simulink model "fuelsys_LN2_breach"  (R2017a)
settings: Solver=ode45  StartTime=0.0  StopTime=tspan(end)  FixedStep=0.001  RelTol=1e-5  AbsTol=1e-6
PostLoadFcn:
  | sldemo_fuelsys_data(bdroot,'initialize_data','orig','float');
model workspace (MAT data in the model file):
  PressEst = [0.806253176324 0.553142316929 0.37151500209 0.277667903103 0.220198954207 0.181288665766 0.153200000489 0.115431020872 0.0913067476324 0.0746519188607 0.0625231108324 0.0533383634277 ... (306 elements, 18x17)]
  PressVect = [0.05 0.1 0.15 0.2 0.25 0.3 0.35 0.4 0.45 0.5 0.55 0.6 0.65 0.7 0.75 0.8 0.85 0.9 0.95]
  PumpCon = [-0.0556348 -0.0022828 0.0256932 0.0435188 0.0562692 0.0661194857143 0.0741572 0.08697 0.0972452 0.106070342857 0.1139892 0.121303866667 ... (342 elements, 18x19)]
  RampRateKiX = [100 200 300 400 500 600]
  RampRateKiY = [0 0.2 0.4 0.6 0.8 1]
  RampRateKiZ = [0.012  0.024  0.036  0.048  0.06  0.072; 0.024  0.048  0.072  0.096  0.12  0.144; 0.036  0.072  0.108  0.144  0.18  0.216; 0.048  0.096  0.144  0.192  0.24  0.288; 0.06  0.12  0.18  0.24  0.3  0.36; 0.072  0.144  0.216  0.288  0.36  0.432]
  SpeedEst = [471.837839721 550.80940091 777.559313277 1080.9243499 1418.36795322 1769.7468768 2125.37309264 2480.20345067 2831.37796793 3177.14006959 3516.32917143 4064.90417867 ... (323 elements, 17x19)]
  SpeedVect = [50 75 100 125 150 175 200 250 300 350 400 450 500 600 700 800 900 1000]
  ThrotEst = [0 0 0 0 0 0 0 0 0 0 0 0 ... (342 elements, 18x19)]
  ThrotVect = [0 3 6 9 12 15 18 21 24 27 30 35 46 57 68 79 90]
  ego_sw = 1
  engine_speed = 300
  hys = 25
  map_sw = 1
  max_ego = 1.2
  max_press = 0.95
  max_speed = 628
  max_throt = 90
  min_press = 0.05
  min_speed = 50
  min_throt = 3
  speed_sw = 1
  st_range = 0.0001
  throttle_sw = 1
  zero_thresh = 250
undefined symbols (not defined in the file): DiscIntNeverNeededParam, sld_FuelModes, sldvsubsys
libraries: simulink x7, simulink_extras x2
(part 1 of 2)
CloseFcn:
  | clear EngSensors u8En* s16En* sldemo_fuelsys_output
Description:
  | This is a model of a fuel control system where Stateflow(R) is used to handle the fault management of the system.
  | The system contains four separate sensors: a throttle sensor, a speed sensor, an oxygen sensor, and a pressure sensor.
  | Each of these sensors is represented by a parallel state in Stateflow.  Each parallel state contains two substates, a
  | normal state and a failed state (the exception being the oxygen sensor, which also contains a warmup state).
  | 
  | If any of the sensor readings is outside an acceptable range, then a fault is registered in Stateflow, and the
  | substate of the corresponding subsystem transitions to the failed state.  If a subsystem recovers, it can
  | transition back to the normal state.  The number of failures in the system at any given time is represented
  | in the Fail parallel state.
  | 
  | The last parallel state in the Stateflow chart is called Fueling_Mode.  This state regulates the oxygen to
  | fuel mixture ratio.  If a failure is detected, then the oxygen to fuel ratio is increased.  If multiple failures
  | are detected, then the fuel system is disabled until there are no longer multiple failures in the system.
settings Model: ModifiedByFormat=The MathWorks Inc.  ExtModeTrigMode=oneshot  ExtModeArmWhenConnect=off  ExtModeAutoUpdateStatusClock=off  Creator=The MathWorks, Inc.  LastModifiedBy=The MathWorks Inc.
settings DataIOCC: ExternalInput=[t__, u__]  LoadExternalInput=on  SaveFormat=StructureWithTime  ReturnWorkspaceOutputs=on
settings OptimizationCC: DefaultParameterBehavior=Inlined  UseDivisionForNetSlopeComputation=UseDivisionForReciprocalsOfIntegersOnly  InlineInvariantSignals=on  EnhancedBackFolding=on  StrengthReduction=on  BooleansAsBitfields=on  PassReuseOutputArgsAs=Individual arguments  ExpressionDepthLimit=2147483647  ZeroExternalMemoryAtStartup=off  ZeroInternalMemoryAtStartup=off  NoFixptDivByZeroProtection=on  EfficientFloat2IntCast=on  LifeSpan=1
settings DebuggingCC: SignalInfNanChecking=error  SaveWithParameterizedLinksMsg=none  UnderspecifiedInitializationDetection=Classic  CheckExecutionContextPreStartOutputMsg=on  CheckExecutionContextRuntimeOutputMsg=on  IntegerOverflowMsg=none  ParameterDowncastMsg=warning  ParameterOverflowMsg=none  ParameterPrecisionLossMsg=none  UnderSpecifiedDataTypeMsg=warning  FcnCallInpInsideContextMsg=warning  UniqueDataStoreMsg=error  BusObjectLabelMismatch=error  StateNameClashWarn=warning  StrictBusMsg=ErrorOnBusTreatedAsVector  SFUnexpectedBacktrackingDiag=warning  SFNoUnconditionalDefaultTransitionDiag=warning  SFExecutionAtInitializationDiag=none  IntegerSaturationMsg=none
settings HardwareCC: ProdBitPerPointer=32  ProdBitPerSizeT=32  ProdBitPerPtrDiffT=32  ProdLargestAtomicFloat=None  ProdWordSize=32  ProdHWDeviceType=Specified
settings ModelReferenceCC: PropagateSignalLabelsOutOfModel=off
settings SFSimCC: SimParseCustomCode=off  MATLABDynamicMemAlloc=off
settings RTWCC: SystemTargetFile=ert.tlc  TemplateMakefile=ert_default_tmf  Description=Real-Time Workshop Embedded Coder  RTWVerbose=off  IncludeHyperlinkInReport=on
settings CodeAppCC: ForceParamTrailComments=on  IgnoreCustomStorageClasses=off  IgnoreTestpoints=on  SimulinkDataObjDesc=on  SFDataObjDesc=on  CustomSymbolStrGlobalVar=rt$N$M  CustomSymbolStrType=$N$M  CustomSymbolStrFcn=$N$M$F  CustomSymbolStrMacro=$N$M  InsertBlockDesc=on  InternalIdentifier=Classic  ReqsInCode=on
settings ERTTargetCC: MultiwordLength=2048  GenerateSampleERTMain=on  IncludeMdlTerminateFcn=off  SupportAbsoluteTime=off  SupportNonFinite=off  SupportComplex=off  InlinedParameterPlacement=NonHierarchical  ERTCustomFileTemplate=example_file_process.tlc  ConvertIfToSwitch=off  SuppressUnreachableDefaultCases=off
settings ConfigComp: CovScope=Subsystem  CovPath=/fuel_rate_control/control_logic  CovMetricSettings=dw  CovHtmlReporting=on  CovSaveCumulativeToWorkspaceVar=on  CovSaveSingleToWorkspaceVar=on  CovExternalEMLEnable=off  CovSFcnEnable=off

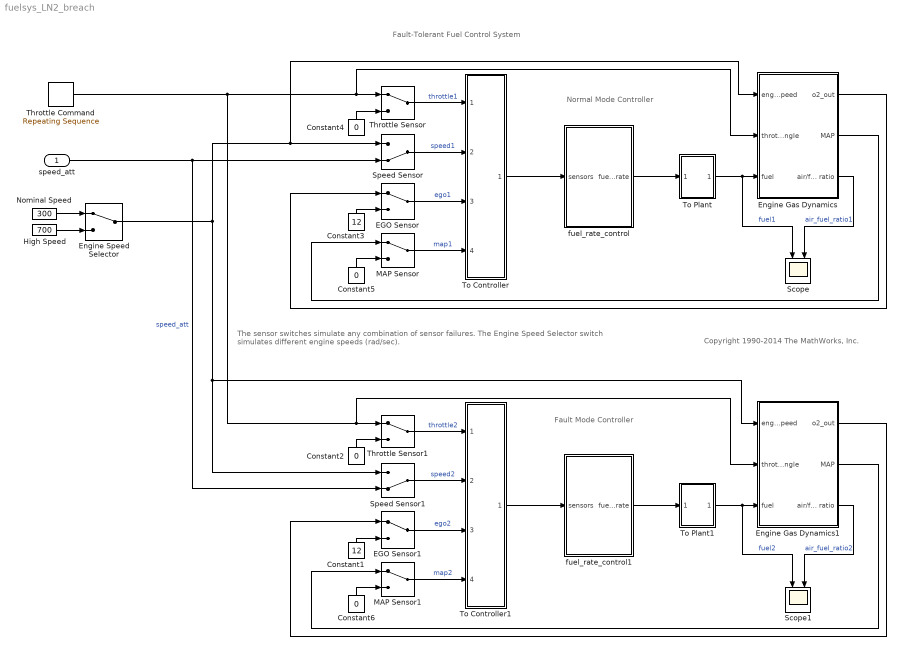
== system fuelsys_LN2_breach ==
  note: Normal Mode Controller
  note: Fault-Tolerant Fuel Control System
  note: Copyright 1990-2014 The MathWorks, Inc.
  note: The sensor switches simulate any combination of sensor failures.
      | The Engine Speed Selector switch simulates different engine speeds (rad/sec).
  note: Fault Mode Controller
  speed_att : Inport
  Constant1 : Constant  Value=12
  Constant{2,4..6} (4 alike) : Constant  Value=0
  Constant3 : Constant  Value=12
  EGO Sensor : ManualSwitch
  EGO Sensor1 : ManualSwitch
  Engine Speed Selector : ManualSwitch
  Engine Gas Dynamics : Subsystem
  Engine Gas Dynamics1 : Subsystem
  High Speed : Constant  Value=700
  MAP Sensor : ManualSwitch
  MAP Sensor1 : ManualSwitch
  Nominal Speed : Constant  Value=300
  Scope : Scope  NumInputPorts=2
  Scope1 : Scope  NumInputPorts=2
  Speed Sensor : ManualSwitch  CurrentSetting=0
  Speed Sensor1 : ManualSwitch  CurrentSetting=0
  Throttle Command : simulink/Sources/Repeating Sequence  rep_seq_t=[0 2 4]  rep_seq_y=[10 20 10]
  Throttle Sensor : ManualSwitch
  Throttle Sensor1 : ManualSwitch
  To Controller : Subsystem
      mask Display: fprintf('Convert')
  To Controller1 : Subsystem
      mask Display: fprintf('Convert')
  To Plant : Subsystem
      mask Display: fprintf('Convert')
  To Plant1 : Subsystem
      mask Display: fprintf('Convert')
  fuel_rate_control : Subsystem  Tag=FuelRateControl  TreatAsAtomicUnit=on
  fuel_rate_control1 : Subsystem  Tag=FuelRateControl  TreatAsAtomicUnit=on
  wires:
  Engine Gas Dynamics/3(air/fuel ratio) -> Scope/2  "air_fuel_ratio1"
  fuel_rate_control/1(fuel_rate) -> To Plant/1(In1)
  Engine Gas Dynamics/1(o2_out) -> EGO Sensor/1
  Constant5/1 -> MAP Sensor/2
  Constant3/1 -> EGO Sensor/2
  Constant4/1 -> Throttle Sensor/2
  Engine Gas Dynamics/2(MAP) -> MAP Sensor/1
  High Speed/1 -> Engine Speed Selector/2
  Nominal Speed/1 -> Engine Speed Selector/1
  EGO Sensor/1 -> To Controller/3(ego)  "ego1"
  MAP Sensor/1 -> To Controller/4(map)  "map1"
  Throttle Sensor/1 -> To Controller/1(throttle)  "throttle1"
  Speed Sensor/1 -> To Controller/2(speed)  "speed1"
  To Plant/1(Out1) -> Scope/1, Engine Gas Dynamics/3(fuel)  "fuel1"
  To Controller/1(sensors) -> fuel_rate_control/1(sensors)
  Engine Gas Dynamics1/3(air/fuel ratio) -> Scope1/2  "air_fuel_ratio2"
  Engine Speed Selector/1 -> Engine Gas Dynamics/1(engine speed), Speed Sensor/1, Engine Gas Dynamics1/1(engine speed), Speed Sensor1/1
  fuel_rate_control1/1(fuel_rate) -> To Plant1/1(In1)
  Engine Gas Dynamics1/1(o2_out) -> EGO Sensor1/1
  Constant6/1 -> MAP Sensor1/2
  Constant1/1 -> EGO Sensor1/2
  Throttle Command/1 -> Engine Gas Dynamics/2(throttle angle), Throttle Sensor/1, Engine Gas Dynamics1/2(throttle angle), Throttle Sensor1/1
  Constant2/1 -> Throttle Sensor1/2
  Engine Gas Dynamics1/2(MAP) -> MAP Sensor1/1
  EGO Sensor1/1 -> To Controller1/3(ego)  "ego2"
  MAP Sensor1/1 -> To Controller1/4(map)  "map2"
  Throttle Sensor1/1 -> To Controller1/1(throttle)  "throttle2"
  Speed Sensor1/1 -> To Controller1/2(speed)  "speed2"
  To Plant1/1(Out1) -> Scope1/1, Engine Gas Dynamics1/3(fuel)  "fuel2"
  To Controller1/1(sensors) -> fuel_rate_control1/1(sensors)
  speed_att/1 -> Speed Sensor1/2, Speed Sensor/2  "speed_att"

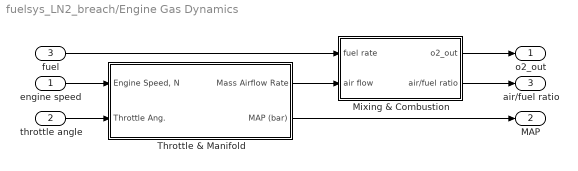
== system fuelsys_LN2_breach/Engine Gas Dynamics ==
  engine speed : Inport
  throttle angle : Inport  Port=2
  fuel : Inport  Port=3
  Mixing & Combustion : Subsystem
  Throttle & Manifold : Subsystem
  o2_out : Outport
  MAP : Outport  Port=2
  air/fuel ratio : Outport  Port=3
  wires:
  Throttle & Manifold/1(Mass Airflow Rate) -> Mixing & Combustion/2(air flow)
  fuel/1 -> Mixing & Combustion/1(fuel rate)
  engine speed/1 -> Throttle & Manifold/1("Engine Speed, N")
  throttle angle/1 -> Throttle & Manifold/2(Throttle Ang.)
  Mixing & Combustion/2(air/fuel ratio) -> air/fuel ratio/1
  Throttle & Manifold/2(MAP (bar)) -> MAP/1
  Mixing & Combustion/1(o2_out) -> o2_out/1

== system fuelsys_LN2_breach/Engine Gas Dynamics1 ==
  engine speed : Inport
  throttle angle : Inport  Port=2
  fuel : Inport  Port=3
  Mixing & Combustion : Subsystem
  Throttle & Manifold : Subsystem
  o2_out : Outport
  MAP : Outport  Port=2
  air/fuel ratio : Outport  Port=3
  wires:
  Throttle & Manifold/1(Mass Airflow Rate) -> Mixing & Combustion/2(air flow)
  fuel/1 -> Mixing & Combustion/1(fuel rate)
  engine speed/1 -> Throttle & Manifold/1("Engine Speed, N")
  throttle angle/1 -> Throttle & Manifold/2(Throttle Ang.)
  Mixing & Combustion/2(air/fuel ratio) -> air/fuel ratio/1
  Throttle & Manifold/2(MAP (bar)) -> MAP/1
  Mixing & Combustion/1(o2_out) -> o2_out/1

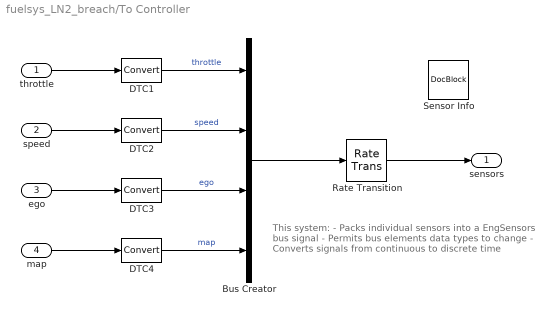
== system fuelsys_LN2_breach/To Controller ==
  note: This system:
      | - Packs individual sensors into a EngSensors bus signal
      | - Permits bus elements data types to change
      | - Converts signals from continuous to discrete time
  throttle : Inport
  speed : Inport  Port=2
  ego : Inport  Port=3
  map : Inport  Port=4
  Bus Creator : BusCreator  Inputs=4  OutDataTypeStr=Bus: EngSensors  NonVirtualBus=on
  DTC{1..4} (4 alike) : DataTypeConversion  SampleTime=[0 1]
  Rate Transition : RateTransition  OutPortSampleTime=0.01
  Sensor Info : simulink/Model-Wide Utilities/DocBlock  DocumentType=Text
      content=|
      | Measurement Descriptions
      | ========================
      |
      | Throttle Angle (degrees):
      | min=3, max=90, precision=0.1
      |
      | Engine Speed (radians/sec.):
      | min=0, max=620, precision=.1
      |
      | Ego Sensor (volts):
      | min=0, max=12, precision=.05
      |
      | Manifold Pressure (bar):
      | min=0.001, max=1, precision=.001
  sensors : Outport
  wires:
  throttle/1 -> DTC1/1
  DTC1/1 -> Bus Creator/1  "throttle"
  speed/1 -> DTC2/1
  DTC2/1 -> Bus Creator/2  "speed"
  ego/1 -> DTC3/1
  DTC3/1 -> Bus Creator/3  "ego"
  map/1 -> DTC4/1
  DTC4/1 -> Bus Creator/4  "map"
  Bus Creator/1 -> Rate Transition/1
  Rate Transition/1 -> sensors/1

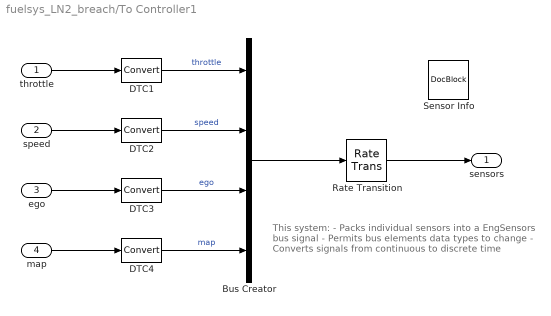
== system fuelsys_LN2_breach/To Controller1 ==
  note: This system:
      | - Packs individual sensors into a EngSensors bus signal
      | - Permits bus elements data types to change
      | - Converts signals from continuous to discrete time
  throttle : Inport
  speed : Inport  Port=2
  ego : Inport  Port=3
  map : Inport  Port=4
  Bus Creator : BusCreator  Inputs=4  OutDataTypeStr=Bus: EngSensors  NonVirtualBus=on
  DTC{1..4} (4 alike) : DataTypeConversion  SampleTime=[0 1]
  Rate Transition : RateTransition  OutPortSampleTime=0.01
  Sensor Info : simulink/Model-Wide Utilities/DocBlock  DocumentType=Text
      content=|
      | Measurement Descriptions
      | ========================
      |
      | Throttle Angle (degrees):
      | min=3, max=90, precision=0.1
      |
      | Engine Speed (radians/sec.):
      | min=0, max=620, precision=.1
      |
      | Ego Sensor (volts):
      | min=0, max=12, precision=.05
      |
      | Manifold Pressure (bar):
      | min=0.001, max=1, precision=.001
  sensors : Outport
  wires:
  throttle/1 -> DTC1/1
  DTC1/1 -> Bus Creator/1  "throttle"
  speed/1 -> DTC2/1
  DTC2/1 -> Bus Creator/2  "speed"
  ego/1 -> DTC3/1
  DTC3/1 -> Bus Creator/3  "ego"
  map/1 -> DTC4/1
  DTC4/1 -> Bus Creator/4  "map"
  Bus Creator/1 -> Rate Transition/1
  Rate Transition/1 -> sensors/1

== system fuelsys_LN2_breach/To Plant ==
  note: This system:
      | - Permits upstream signal data type to change
      | - Converts signals from discrete to continuous time
  In1 : Inport
  DTC5 : DataTypeConversion
  Rate Transition1 : RateTransition  Integrity=off  X0=1.6  OutPortSampleTime=0
  Out1 : Outport
  wires:
  DTC5/1 -> Rate Transition1/1
  In1/1 -> DTC5/1
  Rate Transition1/1 -> Out1/1

== system fuelsys_LN2_breach/To Plant1 ==
  note: This system:
      | - Permits upstream signal data type to change
      | - Converts signals from discrete to continuous time
  In1 : Inport
  DTC5 : DataTypeConversion
  Rate Transition1 : RateTransition  Integrity=off  X0=1.6  OutPortSampleTime=0
  Out1 : Outport
  wires:
  DTC5/1 -> Rate Transition1/1
  In1/1 -> DTC5/1
  Rate Transition1/1 -> Out1/1

== system fuelsys_LN2_breach/fuel_rate_control ==
  note: Fuel Rate Control Subsystem
  sensors : Inport  OutDataTypeStr=Bus: EngSensors
  Bus Selector1 : BusSelector  OutputSignals=speed
  airflow_calc : Subsystem
  control_logic : Stateflow chart  Description=Stateflow diagram to determine control system operating mode  TreatAsAtomicUnit=on
  fuel_calc : Subsystem
  validate_sample_time : Subsystem  Tag=VerificationSubsystem  DisableCoverage=on  LoadFcn=sldvsubsys('check')  TreatAsAtomicUnit=on  SimViewingDevice=on  mask(VerificationSubsystem){}
      mask init:
      | sldvsubsys('maskInit');
      settings: CopyFcn=sldvsubsys('copy');  OpenFcn=open_system(gcb,'force');
      settings: PreSaveFcn=|
      | set_param(gcb,'SimViewingDevice','on');
      | sldvsubsys('check');
      mask Help: helpview(fullfile(docroot,'toolbox','sldv','sldv.map'),'verificationsubsystem')
      mask Display: image(imread('sldvicon_versubsys.png','BackGroundColor',[1 1 1]),'center');
  fuel_rate : Outport
  wires:
  fuel_calc/1(fuel_rate) -> fuel_rate/1
  airflow_calc/1(est_airflow) -> fuel_calc/1(est_airflow)
  sensors/1 -> control_logic/1(es_i), Bus Selector1/1
  control_logic/3(fuel_mode) -> airflow_calc/3(fuel_mode), fuel_calc/3(fuel_mode)
  control_logic/1(es_o) -> airflow_calc/1(sensors)
  control_logic/2(" O2_normal") -> airflow_calc/2(O2_normal)
  airflow_calc/2(fb_correction) -> fuel_calc/2(fb_correction)
  Bus Selector1/1 -> validate_sample_time/1(In1)  "<speed>"

== system fuelsys_LN2_breach/fuel_rate_control1 ==
  note: Fuel Rate Control Subsystem
  sensors : Inport  OutDataTypeStr=Bus: EngSensors
  Bus Selector1 : BusSelector  OutputSignals=speed
  airflow_calc : Subsystem
  control_logic : Stateflow chart  Description=Stateflow diagram to determine control system operating mode  TreatAsAtomicUnit=on
  fuel_calc : Subsystem
  validate_sample_time : Subsystem  Tag=VerificationSubsystem  DisableCoverage=on  LoadFcn=sldvsubsys('check')  TreatAsAtomicUnit=on  SimViewingDevice=on  mask(VerificationSubsystem){}
      mask init:
      | sldvsubsys('maskInit');
      settings: CopyFcn=sldvsubsys('copy');  OpenFcn=open_system(gcb,'force');
      settings: PreSaveFcn=|
      | set_param(gcb,'SimViewingDevice','on');
      | sldvsubsys('check');
      mask Help: helpview(fullfile(docroot,'toolbox','sldv','sldv.map'),'verificationsubsystem')
      mask Display: image(imread('sldvicon_versubsys.png','BackGroundColor',[1 1 1]),'center');
  fuel_rate : Outport
  wires:
  fuel_calc/1(fuel_rate) -> fuel_rate/1
  airflow_calc/1(est_airflow) -> fuel_calc/1(est_airflow)
  sensors/1 -> control_logic/1(es_i), Bus Selector1/1
  control_logic/3(fuel_mode) -> airflow_calc/3(fuel_mode), fuel_calc/3(fuel_mode)
  control_logic/1(es_o) -> airflow_calc/1(sensors)
  control_logic/2(" O2_normal") -> airflow_calc/2(O2_normal)
  airflow_calc/2(fb_correction) -> fuel_calc/2(fb_correction)
  Bus Selector1/1 -> validate_sample_time/1(In1)  "<speed>"

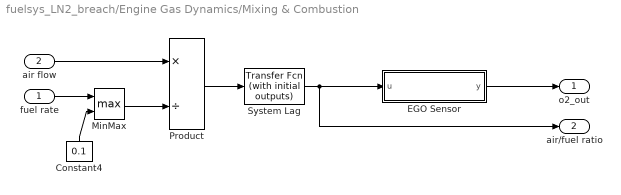
== system fuelsys_LN2_breach/Engine Gas Dynamics/Mixing & Combustion ==
  fuel rate : Inport
  air flow : Inport  Port=2
  Constant4 : Constant  Value=0.1
  EGO Sensor : MATLAB Function  TreatAsAtomicUnit=on
  MinMax : MinMax  Function=max  Inputs=2  SaturateOnIntegerOverflow=on  InputSameDT=on
  Product : Product  Inputs=*/  SaturateOnIntegerOverflow=on  RndMeth=Zero  InputSameDT=on  OutDataTypeStr=Inherit: Same as first input
  System Lag : simulink_extras/Additional Linear/Transfer Fcn (with initial outputs)  N=3  D=[1 3]  Y0=1/14.6  U0=1/14.6
  o2_out : Outport
  air/fuel ratio : Outport  Port=2
  wires:
  Constant4/1 -> MinMax/2
  fuel rate/1 -> MinMax/1
  MinMax/1 -> Product/2
  Product/1 -> System Lag/1
  System Lag/1 -> air/fuel ratio/1, EGO Sensor/1(u)
  EGO Sensor/1(y) -> o2_out/1
  air flow/1 -> Product/1

== system fuelsys_LN2_breach/Engine Gas Dynamics/Throttle & Manifold ==
  note: Air-Fuel Intake Dynamics
  "Engine Speed, N" : Inport
  Throttle Ang. : Inport  Port=2
  "Atmospheric Pressure, Pa (bar)" : Constant  Value=1.0
  Intake Manifold : Subsystem
  Limit to Positive : Saturate  UpperLimit=inf  LowerLimit=0
  Throttle : Subsystem
  Mass Airflow Rate : Outport
  MAP (bar) : Outport  Port=2
  wires:
  Limit to Positive/1 -> Throttle/1("Throttle Angle, theta (deg)")
  Throttle Ang./1 -> Limit to Positive/1
  Throttle/1("Throttle Flow, mdot (g/s)") -> Intake Manifold/1(mdot Input (g/s))
  "Engine Speed, N"/1 -> Intake Manifold/2(N (rad/sec))
  Intake Manifold/1(mdot to Cylinder (g/s)) -> Mass Airflow Rate/1
  "Atmospheric Pressure, Pa (bar)"/1 -> Throttle/3("Atmospheric Pressure, Pa (bar) ")
  Intake Manifold/2("Manifold Pressure, Pm (bar)") -> Throttle/2("Manifold Pressure, Pm (bar)"), MAP (bar)/1

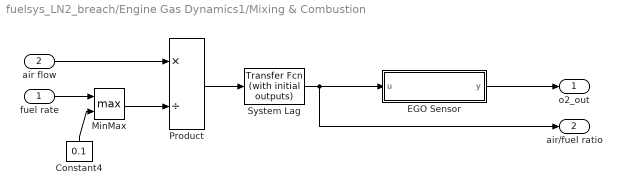
== system fuelsys_LN2_breach/Engine Gas Dynamics1/Mixing & Combustion ==
  fuel rate : Inport
  air flow : Inport  Port=2
  Constant4 : Constant  Value=0.1
  EGO Sensor : MATLAB Function  TreatAsAtomicUnit=on
  MinMax : MinMax  Function=max  Inputs=2  SaturateOnIntegerOverflow=on  InputSameDT=on
  Product : Product  Inputs=*/  SaturateOnIntegerOverflow=on  RndMeth=Zero  InputSameDT=on  OutDataTypeStr=Inherit: Same as first input
  System Lag : simulink_extras/Additional Linear/Transfer Fcn (with initial outputs)  N=3  D=[1 3]  Y0=1/14.6  U0=1/14.6
  o2_out : Outport
  air/fuel ratio : Outport  Port=2
  wires:
  Constant4/1 -> MinMax/2
  fuel rate/1 -> MinMax/1
  MinMax/1 -> Product/2
  Product/1 -> System Lag/1
  System Lag/1 -> air/fuel ratio/1, EGO Sensor/1(u)
  EGO Sensor/1(y) -> o2_out/1
  air flow/1 -> Product/1

== system fuelsys_LN2_breach/Engine Gas Dynamics1/Throttle & Manifold ==
  note: Air-Fuel Intake Dynamics
  "Engine Speed, N" : Inport
  Throttle Ang. : Inport  Port=2
  "Atmospheric Pressure, Pa (bar)" : Constant  Value=1.0
  Intake Manifold : Subsystem
  Limit to Positive : Saturate  UpperLimit=inf  LowerLimit=0
  Throttle : Subsystem
  Mass Airflow Rate : Outport
  MAP (bar) : Outport  Port=2
  wires:
  Limit to Positive/1 -> Throttle/1("Throttle Angle, theta (deg)")
  Throttle Ang./1 -> Limit to Positive/1
  Throttle/1("Throttle Flow, mdot (g/s)") -> Intake Manifold/1(mdot Input (g/s))
  "Engine Speed, N"/1 -> Intake Manifold/2(N (rad/sec))
  Intake Manifold/1(mdot to Cylinder (g/s)) -> Mass Airflow Rate/1
  "Atmospheric Pressure, Pa (bar)"/1 -> Throttle/3("Atmospheric Pressure, Pa (bar) ")
  Intake Manifold/2("Manifold Pressure, Pm (bar)") -> Throttle/2("Manifold Pressure, Pm (bar)"), MAP (bar)/1

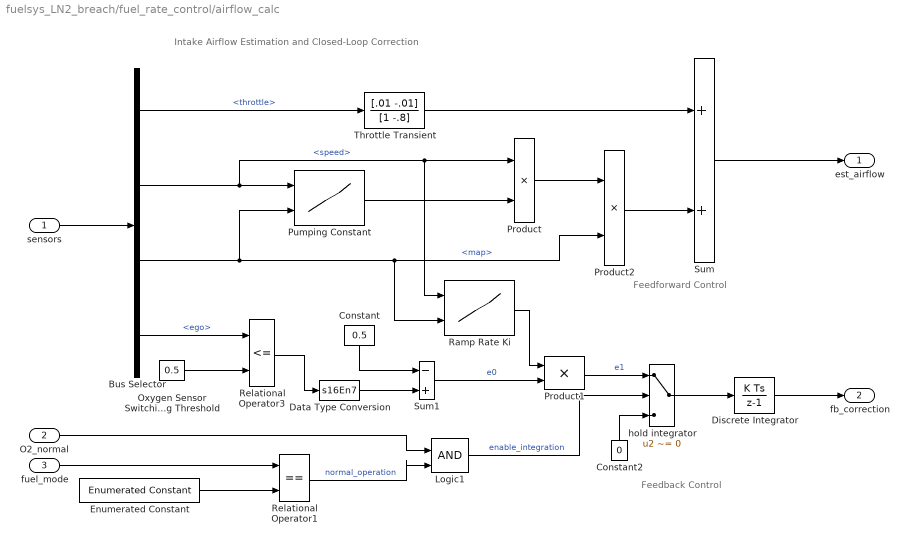
== system fuelsys_LN2_breach/fuel_rate_control/airflow_calc ==
  note: Intake Airflow Estimation and Closed-Loop Correction
  note: Feedback Control
  note: Feedforward Control
  sensors : Inport
  O2_normal : Inport  Port=2
  fuel_mode : Inport  Port=3
  Bus Selector : BusSelector  OutputSignals=throttle,speed,map,ego
  Constant : Constant  Value=0.5  OutDataTypeStr=s16En7
  Constant2 : Constant  Value=0  OutDataTypeStr=uint8
  Data Type Conversion : DataTypeConversion  OutDataTypeStr=s16En7  RndMeth=Simplest
  Discrete Integrator : DiscreteIntegrator  InitialConditionSetting=State (most efficient)  SampleTime=-1  OutDataTypeStr=s16En15  RndMeth=Simplest  ICPrevOutput=DiscIntNeverNeededParam  ICPrevScaledInput=DiscIntNeverNeededParam
  Enumerated Constant : simulink/Sources/Enumerated Constant  OutDataTypeStr=Enum: sld_FuelModes  Value=sld_FuelModes.LOW  SampleTime=.01
      settings: SourceProductName=Simulink
  Logic1 : Logic  IconShape=distinctive  AllPortsSameDT=off  OutDataTypeStr=boolean
  Oxygen Sensor Switching Threshold : Constant  Value=0.5  OutDataTypeStr=s16En7
  Product : Product  OutDataTypeStr=s16En7  RndMeth=Simplest
  Product1 : Product  OutDataTypeStr=s16En15  RndMeth=Simplest
  Product2 : Product  OutDataTypeStr=s16En7  RndMeth=Simplest
  Pumping Constant : Lookup_n-D  BreakpointsForDimension1=SpeedVect  BreakpointsForDimension2=PressVect  IndexSearchMethod=Linear search  Table=PumpCon  ExtrapMethod=Clip  UseLastTableValue=on  OutDataTypeStr=s16En15  RndMeth=Simplest
  Ramp Rate Ki : Lookup_n-D  BreakpointsForDimension1=RampRateKiX  BreakpointsForDimension2=RampRateKiY  IndexSearchMethod=Linear search  Table=RampRateKiZ  ExtrapMethod=Clip  UseLastTableValue=on  OutDataTypeStr=s16En15  RndMeth=Simplest
  Relational Operator1 : RelationalOperator  Operator===  OutDataTypeStr=boolean  RndMeth=Nearest  InputSameDT=on
  Relational Operator3 : RelationalOperator  Operator=<=  OutDataTypeStr=boolean  RndMeth=Nearest
  Sum : Sum  Inputs=2  OutDataTypeStr=s16En7  RndMeth=Simplest
  Sum1 : Sum  Inputs=-+  OutDataTypeStr=s16En15  RndMeth=Simplest
  Throttle Transient : DiscreteFilter  Numerator=[.01 -.01]  Denominator=[1 -.8]  a0EqualsOne=on  OutDataTypeStr=s16En7  RndMeth=Simplest
  hold integrator : Switch  Criteria=u2 ~= 0  Threshold=1  OutDataTypeStr=s16En15  RndMeth=Simplest
  est_airflow : Outport
  fb_correction : Outport  Port=2
  wires:
  Discrete Integrator/1 -> fb_correction/1
  sensors/1 -> Bus Selector/1
  Pumping Constant/1 -> Product/2
  Bus Selector/2 -> Product/1, Ramp Rate Ki/1, Pumping Constant/1  "<speed>"
  Throttle Transient/1 -> Sum/1
  Sum/1 -> est_airflow/1
  Bus Selector/1 -> Throttle Transient/1  "<throttle>"
  Relational Operator1/1 -> Logic1/2  "normal_operation"
  Oxygen Sensor Switching Threshold/1 -> Relational Operator3/2
  Constant/1 -> Sum1/1
  Ramp Rate Ki/1 -> Product1/1
  Constant2/1 -> hold integrator/3
  Product1/1 -> hold integrator/1  "e1"
  hold integrator/1 -> Discrete Integrator/1
  Logic1/1 -> hold integrator/2  "enable_integration"
  Sum1/1 -> Product1/2  "e0"
  Relational Operator3/1 -> Data Type Conversion/1
  Data Type Conversion/1 -> Sum1/2
  Bus Selector/3 -> Product2/2, Ramp Rate Ki/2, Pumping Constant/2  "<map>"
  Bus Selector/4 -> Relational Operator3/1  "<ego>"
  Product/1 -> Product2/1
  Product2/1 -> Sum/2
  O2_normal/1 -> Logic1/1
  Enumerated Constant/1 -> Relational Operator1/2
  fuel_mode/1 -> Relational Operator1/1

== system fuelsys_LN2_breach/fuel_rate_control/control_logic/Pressure.map_estimate ==
  note: MAP Estimation
  speed : Inport  OutDataTypeStr=s16En3
  throttle : Inport  Port=2  OutDataTypeStr=s16En3
  f : TriggerPort  TriggerType=function-call  VariantControl=Variant
      settings: CopyFcn=Stateflow.SLINSF.SimulinkMan.removeBlockPreDeleteFcn  PreDeleteFcn=Stateflow.SLINSF.SimulinkMan.unsafePredeleteFcn
  Pressure Estimation : Lookup_n-D  BreakpointsForDimension1=SpeedVect  BreakpointsForDimension2=ThrotVect  IndexSearchMethod=Linear search  Table=PressEst  ExtrapMethod=Clip  UseLastTableValue=on  OutDataTypeStr=u8En7  RndMeth=Simplest
  map : Outport
  wires:
  speed/1 -> Pressure Estimation/1
  throttle/1 -> Pressure Estimation/2
  Pressure Estimation/1 -> map/1

== system fuelsys_LN2_breach/fuel_rate_control/control_logic/Speed.speed_estimate ==
  note: Speed Estimation
  throttle : Inport  OutDataTypeStr=s16En3
  map : Inport  Port=2  OutDataTypeStr=u8En7
  f : TriggerPort  TriggerType=function-call  VariantControl=Variant
      settings: CopyFcn=Stateflow.SLINSF.SimulinkMan.removeBlockPreDeleteFcn  PreDeleteFcn=Stateflow.SLINSF.SimulinkMan.unsafePredeleteFcn
  Saturation : Saturate  UpperLimit=max_speed  LowerLimit=0  OutDataTypeStr=s16En3
  Speed Estimation : Lookup_n-D  BreakpointsForDimension1=ThrotVect  BreakpointsForDimension2=PressVect  IndexSearchMethod=Linear search  Table=SpeedEst  ExtrapMethod=Clip  UseLastTableValue=on  OutDataTypeStr=s16En3  RndMeth=Simplest
  speed : Outport
  wires:
  Speed Estimation/1 -> Saturation/1
  throttle/1 -> Speed Estimation/1
  map/1 -> Speed Estimation/2
  Saturation/1 -> speed/1

== system fuelsys_LN2_breach/fuel_rate_control/control_logic/Throttle.throttle_estimate ==
  note: Throttle Estimation
  speed : Inport  OutDataTypeStr=s16En3
  map : Inport  Port=2  OutDataTypeStr=u8En7
  f : TriggerPort  TriggerType=function-call  VariantControl=Variant
      settings: CopyFcn=Stateflow.SLINSF.SimulinkMan.removeBlockPreDeleteFcn  PreDeleteFcn=Stateflow.SLINSF.SimulinkMan.unsafePredeleteFcn
  Throttle Estimation : Lookup_n-D  BreakpointsForDimension1=SpeedVect  BreakpointsForDimension2=PressVect  IndexSearchMethod=Linear search  Table=ThrotEst  ExtrapMethod=Clip  UseLastTableValue=on  OutDataTypeStr=s16En7  RndMeth=Simplest
  throttle : Outport
  wires:
  speed/1 -> Throttle Estimation/1
  map/1 -> Throttle Estimation/2
  Throttle Estimation/1 -> throttle/1

== system fuelsys_LN2_breach/fuel_rate_control/fuel_calc ==
  note: Fuel Rate Calculation
  est_airflow : Inport
  fb_correction : Inport  Port=2
  fuel_mode : Inport  Port=3
  feedforward_fuel_rate : Subsystem
  switchable_compensation : Subsystem
  fuel_rate : Outport
  wires:
  est_airflow/1 -> feedforward_fuel_rate/1(est_airflow)
  fuel_mode/1 -> feedforward_fuel_rate/2(fuel_mode), switchable_compensation/2(fuel_mode)
  switchable_compensation/1(fuel_rate) -> fuel_rate/1
  fb_correction/1 -> switchable_compensation/3(fb_correction)
  feedforward_fuel_rate/1(ff_fuel_rate) -> switchable_compensation/1(ff_fuel_rate)

== system fuelsys_LN2_breach/fuel_rate_control/validate_sample_time ==
  note: The contents of this subsystem are excluded from the code Simulink Coder generates.
      |
      | To work correctly this system must continue to
      | * Contain no output ports
      | * Enable its 'Treat as Atomic Unit' parameter
      | * Specify its 'Mask type' parameter as "VerificationSubsystem"
  note: Verify sample time: aspects of the design
      | assume a 0.01 second sample time.
  In1 : Inport
  Actual Sample Time : Probe  ProbeWidth=off  ProbeComplexSignal=off  ProbeSampleTimeDataType=Same as input
  CheckRange : simulink/Model Verification/Check  Static Range  Description=-st_range < u < st_range  max=st_range  max_included=off  min=-st_range  min_included=off  enabled=on  stopWhenAssertionFail=on  export=off  icon=graphic
      settings: SourceProductName=Simulink  SourceProductBaseCode=SL
  Data Type Conversion : DataTypeConversion  OutDataTypeStr=s16En15
  Demux : Demux  Outputs=2
  Expected Sample Time : Constant  Value=0.01  OutDataTypeStr=s16En15
  Sum : Sum  Inputs=|+-  OutDataTypeStr=Inherit: Same as first input
  Terminator : Terminator
  wires:
  Actual Sample Time/1 -> Demux/1
  In1/1 -> Data Type Conversion/1
  Demux/2 -> Terminator/1
  Demux/1 -> Sum/1
  Expected Sample Time/1 -> Sum/2
  Sum/1 -> CheckRange/1
  Data Type Conversion/1 -> Actual Sample Time/1

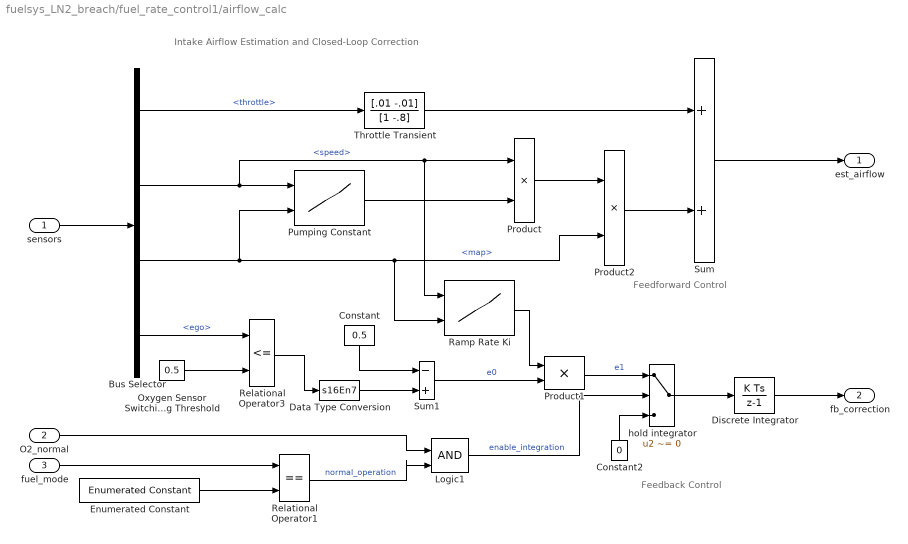
== system fuelsys_LN2_breach/fuel_rate_control1/airflow_calc ==
  note: Intake Airflow Estimation and Closed-Loop Correction
  note: Feedback Control
  note: Feedforward Control
  sensors : Inport
  O2_normal : Inport  Port=2
  fuel_mode : Inport  Port=3
  Bus Selector : BusSelector  OutputSignals=throttle,speed,map,ego
  Constant : Constant  Value=0.5  OutDataTypeStr=s16En7
  Constant2 : Constant  Value=0  OutDataTypeStr=uint8
  Data Type Conversion : DataTypeConversion  OutDataTypeStr=s16En7  RndMeth=Simplest
  Discrete Integrator : DiscreteIntegrator  InitialConditionSetting=State (most efficient)  SampleTime=-1  OutDataTypeStr=s16En15  RndMeth=Simplest  ICPrevOutput=DiscIntNeverNeededParam  ICPrevScaledInput=DiscIntNeverNeededParam
  Enumerated Constant : simulink/Sources/Enumerated Constant  OutDataTypeStr=Enum: sld_FuelModes  Value=sld_FuelModes.LOW  SampleTime=.01
      settings: SourceProductName=Simulink
  Logic1 : Logic  IconShape=distinctive  AllPortsSameDT=off  OutDataTypeStr=boolean
  Oxygen Sensor Switching Threshold : Constant  Value=0.5  OutDataTypeStr=s16En7
  Product : Product  OutDataTypeStr=s16En7  RndMeth=Simplest
  Product1 : Product  OutDataTypeStr=s16En15  RndMeth=Simplest
  Product2 : Product  OutDataTypeStr=s16En7  RndMeth=Simplest
  Pumping Constant : Lookup_n-D  BreakpointsForDimension1=SpeedVect  BreakpointsForDimension2=PressVect  IndexSearchMethod=Linear search  Table=PumpCon  ExtrapMethod=Clip  UseLastTableValue=on  OutDataTypeStr=s16En15  RndMeth=Simplest
  Ramp Rate Ki : Lookup_n-D  BreakpointsForDimension1=RampRateKiX  BreakpointsForDimension2=RampRateKiY  IndexSearchMethod=Linear search  Table=RampRateKiZ  ExtrapMethod=Clip  UseLastTableValue=on  OutDataTypeStr=s16En15  RndMeth=Simplest
  Relational Operator1 : RelationalOperator  Operator===  OutDataTypeStr=boolean  RndMeth=Nearest  InputSameDT=on
  Relational Operator3 : RelationalOperator  Operator=<=  OutDataTypeStr=boolean  RndMeth=Nearest
  Sum : Sum  Inputs=2  OutDataTypeStr=s16En7  RndMeth=Simplest
  Sum1 : Sum  Inputs=-+  OutDataTypeStr=s16En15  RndMeth=Simplest
  Throttle Transient : DiscreteFilter  Numerator=[.01 -.01]  Denominator=[1 -.8]  a0EqualsOne=on  OutDataTypeStr=s16En7  RndMeth=Simplest
  hold integrator : Switch  Criteria=u2 ~= 0  Threshold=1  OutDataTypeStr=s16En15  RndMeth=Simplest
  est_airflow : Outport
  fb_correction : Outport  Port=2
  wires:
  Discrete Integrator/1 -> fb_correction/1
  sensors/1 -> Bus Selector/1
  Pumping Constant/1 -> Product/2
  Bus Selector/2 -> Product/1, Ramp Rate Ki/1, Pumping Constant/1  "<speed>"
  Throttle Transient/1 -> Sum/1
  Sum/1 -> est_airflow/1
  Bus Selector/1 -> Throttle Transient/1  "<throttle>"
  Relational Operator1/1 -> Logic1/2  "normal_operation"
  Oxygen Sensor Switching Threshold/1 -> Relational Operator3/2
  Constant/1 -> Sum1/1
  Ramp Rate Ki/1 -> Product1/1
  Constant2/1 -> hold integrator/3
  Product1/1 -> hold integrator/1  "e1"
  hold integrator/1 -> Discrete Integrator/1
  Logic1/1 -> hold integrator/2  "enable_integration"
  Sum1/1 -> Product1/2  "e0"
  Relational Operator3/1 -> Data Type Conversion/1
  Data Type Conversion/1 -> Sum1/2
  Bus Selector/3 -> Product2/2, Ramp Rate Ki/2, Pumping Constant/2  "<map>"
  Bus Selector/4 -> Relational Operator3/1  "<ego>"
  Product/1 -> Product2/1
  Product2/1 -> Sum/2
  O2_normal/1 -> Logic1/1
  Enumerated Constant/1 -> Relational Operator1/2
  fuel_mode/1 -> Relational Operator1/1

== system fuelsys_LN2_breach/fuel_rate_control1/control_logic/Pressure.map_estimate ==
  note: MAP Estimation
  speed : Inport  OutDataTypeStr=s16En3
  throttle : Inport  Port=2  OutDataTypeStr=s16En3
  f : TriggerPort  TriggerType=function-call  VariantControl=Variant
      settings: CopyFcn=Stateflow.SLINSF.SimulinkMan.removeBlockPreDeleteFcn  PreDeleteFcn=Stateflow.SLINSF.SimulinkMan.unsafePredeleteFcn
  Pressure Estimation : Lookup_n-D  BreakpointsForDimension1=SpeedVect  BreakpointsForDimension2=ThrotVect  IndexSearchMethod=Linear search  Table=PressEst  ExtrapMethod=Clip  UseLastTableValue=on  OutDataTypeStr=u8En7  RndMeth=Simplest
  map : Outport
  wires:
  speed/1 -> Pressure Estimation/1
  throttle/1 -> Pressure Estimation/2
  Pressure Estimation/1 -> map/1
